simulink model "vrbounce_test"  (R2020a)
settings: Solver=VariableStepAuto  StartTime=0.0  StopTime=Inf  RelTol=1e-3
libraries: vrlib x2
settings Model: Creator=tomoffat  LastModifiedBy=tomoffat

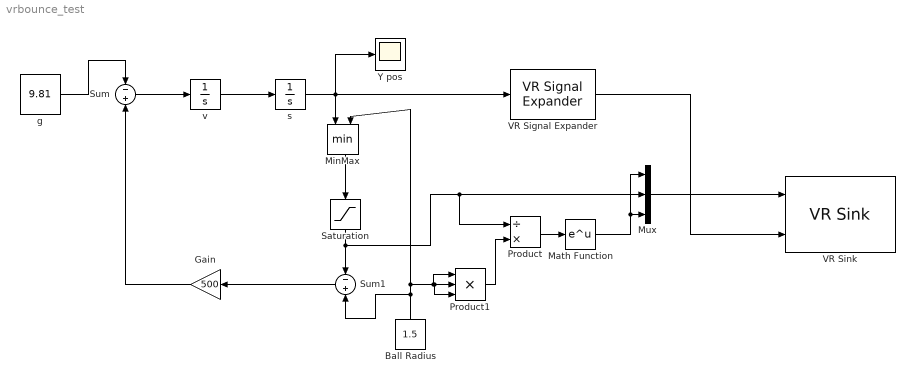
== system vrbounce_test ==
  Ball Radius : Constant  Value=1.5
  Gain : Gain  Gain=500  SaturateOnIntegerOverflow=on  OutDataTypeStr=Inherit: Same as input  ParamDataTypeStr=Inherit: Same as input
  Math Function : Math  SaturateOnIntegerOverflow=on
  MinMax : MinMax  Inputs=2  InputSameDT=on  SaturateOnIntegerOverflow=on
  Mux : Mux  Inputs=3
  Product : Product  Inputs=/*  InputSameDT=on  SaturateOnIntegerOverflow=on  OutDataTypeStr=Inherit: Same as first input
  Product1 : Product  Inputs=3  InputSameDT=on  SaturateOnIntegerOverflow=on  OutDataTypeStr=Inherit: Same as first input
  Saturation : Saturate  UpperLimit=Inf  LowerLimit=1e-4  ZeroCross=off
  Sum : Sum  Inputs=-+  InputSameDT=on  SaturateOnIntegerOverflow=on  OutDataTypeStr=Inherit: Same as first input
  Sum1 : Sum  Inputs=-+  InputSameDT=on  SaturateOnIntegerOverflow=on  OutDataTypeStr=Inherit: Same as first input
  VR Signal Expander : vrlib/VR Signal Expander  outwidth=3  outidx=2
  VR Sink : vrlib/VR Sink  InstantiateOnLoad=on  SampleTime=0.1  ViewEnable=on  RemoteChange=off  RemoteView=off  FieldsWritten=Ball.scale.3.1.1.double#Ball.translation.3.1.1.double  WorldFileName=vrbounce_test.x3d  WorldDescription=VR Bouncing Ball Attempt  AutoView=on  VideoDimensions=[]  AllowVariableSize=off  FigureProperties="{'Position', 'Name', 'Viewpoint', 'CameraBound', 'CameraDirection', 'CameraPosition', 'CameraUpVector', 'ZoomFactor', 'Antialiasing', 'Headlight', 'Lighting', 'NavPanel', 'Sound', 'StatusBar', 'Stereo3D', 'Stereo3DCameraOffset', 'Stereo3DHIT', 'ToolBar', 'Textures', 'Transparency', 'Triad', 'Wireframe', 'NavZones', 'NavMode', 'NavSpeed', 'CaptureFileFormat', 'CaptureFileName', 'Record2DCompressMethod', 'Record2DCompressQuality', 'Record2D', 'Record2DFileName', 'Record2DFPS'; [2.2590000000000000e+03  -2.6500000000000000e+02   5.7600000000000000e+02   3.5000000000000000e+02], 'VR Bouncing Ball Attempt', 'ball', 'on', [0.0000000000000000e+00   0.0000000000000000e+00  -1.0000000000000000e+00], [0.0000000000000000e+00   0.0000000000000000e+00   0.0000000000000000e+00], [0.0000000000000000e+00   1.0000000000000000e+00   0.0000000000000000e+00], [1.0000000000000000e+00], 'on', 'on', 'on', 'halfbar', 'on', 'on', 'off', [1.0000000149011612e-01], [0.0000000000000000e+00], 'on', 'on', 'on', 'none', 'off', 'off', 'examine', 'normal', 'tif', '%f_anim_%n.tif', 'auto', [7.5000000000000000e+01], 'off', '%f_anim_%n.avi', 'auto'}"
  Y pos : Scope
  g : Constant  Value=9.81
  s : Integrator  InitialCondition=20  ZeroCross=off
  v : Integrator  ZeroCross=off
  wires:
  g/1 -> Sum/1
  Sum/1 -> v/1
  v/1 -> s/1
  s/1 -> VR Signal Expander/1, Y pos/1, MinMax/1
  VR Signal Expander/1 -> VR Sink/2
  MinMax/1 -> Saturation/1
  Mux/1 -> VR Sink/1
  Saturation/1 -> Mux/2, Product/1, Sum1/1
  Math Function/1 -> Mux/1, Mux/3
  Product/1 -> Math Function/1
  Ball Radius/1 -> Sum1/2, Product1/1, Product1/3, Product1/2, MinMax/2
  Product1/1 -> Product/2
  Sum1/1 -> Gain/1
  Gain/1 -> Sum/2
